simulink model "v3_sim_sf_sigma_r"  (R2023b)
settings: Solver=VariableStepAuto  StartTime=0.0  StopTime=100  RelTol=1e-10
libraries: simulink x2
settings Model: Creator=kiraa  LastModifiedBy=kiraa

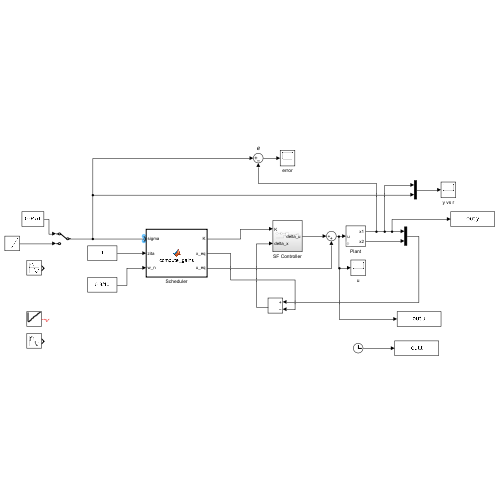
[thumbnail: Simulink's stored preview of the top-level diagram]
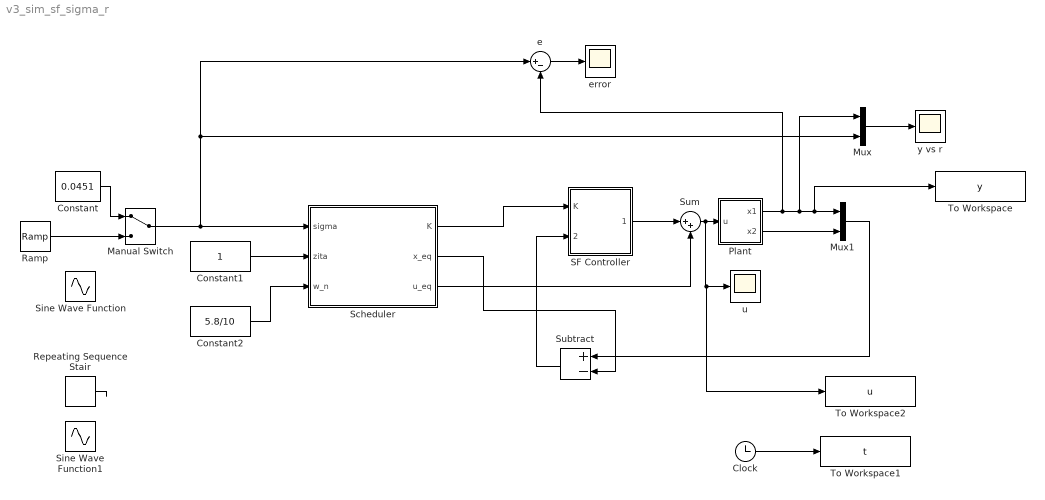
== system v3_sim_sf_sigma_r ==
  Clock : Clock
  Constant : Constant  Value=0.0451
  Constant1 : Constant
  Constant2 : Constant  Value=5.8/10
  Manual Switch : ManualSwitch
  Mux : Mux  Inputs=2
  Mux1 : Mux  Inputs=2
  Plant : Subsystem  mask{x1_0=0.1, x2_0=0}
      mask prompts: x1_0 "x1(0) [g/l]"; x2_0 "x2(0) [min^-1]"
  Ramp : simulink/Sources/Ramp  slope=-0.0005  start=0  InitialOutput=0.1
  Repeating Sequence Stair : simulink/Sources/Repeating Sequence Stair  OutValues=[0.1 0.2 0.3 0.4 0.5 0.6 0.7 0.8 0.9].'  tsamp=20  OutMin=[]  OutMax=[]  OutDataTypeStr=double  OutputDataTypeScalingMode=double  OutDataType=fixdt(0,8)  ConRadixGroup=Best Precision: Vector-wise  OutScaling=2^-12
  SF Controller : Subsystem
  Scheduler : MATLAB Function  TreatAsAtomicUnit=on
  Sine Wave Function : Sin  Amplitude=0.02  Bias=0.05  Frequency=0.1  SampleTime=0
  Sine Wave Function1 : Sin  Amplitude=0.001  Bias=0.0451  Frequency=0.1  Samples=1  SampleTime=2
  Subtract : Sum  Inputs=+-
  Sum : Sum  Inputs=|++
  To Workspace : ToWorkspace  VariableName=y  SampleTime=-1
  To Workspace1 : ToWorkspace  VariableName=t  SampleTime=-1
  To Workspace2 : ToWorkspace  VariableName=u  SampleTime=-1
  e : Sum  Inputs=|+-
  error : Scope
  u : Scope
  y vs r : Scope
  wires:
  Plant/1(x1) -> To Workspace/1, Mux1/1, Mux/1, e/2
  Mux/1 -> y vs r/1
  Constant/1 -> Manual Switch/1
  Manual Switch/1 -> Mux/2, e/1, Scheduler/1(sigma)
  SF Controller/1(delta_u) -> Sum/1
  e/1 -> error/1
  Sum/1 -> To Workspace2/1, u/1, Plant/1(u)
  Scheduler/3(u_eq) -> Sum/2
  Scheduler/1(K) -> SF Controller/1(K)
  Subtract/1 -> SF Controller/2(delta_x)
  Plant/2(x2) -> Mux1/2
  Mux1/1 -> Subtract/1
  Scheduler/2(x_eq) -> Subtract/2
  Constant2/1 -> Scheduler/3(w_n)
  Constant1/1 -> Scheduler/2(zita)
  Repeating Sequence Stair/1 -> ?
  Clock/1 -> To Workspace1/1
  Ramp/1 -> Manual Switch/2

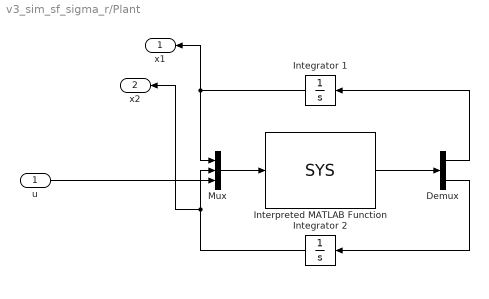
== system v3_sim_sf_sigma_r/Plant ==
  u : Inport
  Demux : Demux  Outputs=2
  Integrator 1 : Integrator  InitialCondition=x1_0
  Integrator 2 : Integrator  InitialCondition=x2_0
  Interpreted MATLAB Function : MATLABFcn  MATLABFcn=SYS  OutputDimensions=2
  Mux : Mux  Inputs=3
  x1 : Outport
  x2 : Outport  Port=2
  wires:
  Integrator 1/1 -> x1/1, Mux/1
  Demux/1 -> Integrator 1/1
  Mux/1 -> Interpreted MATLAB Function/1
  Integrator 2/1 -> x2/1, Mux/2
  Interpreted MATLAB Function/1 -> Demux/1
  Demux/2 -> Integrator 2/1
  u/1 -> Mux/3

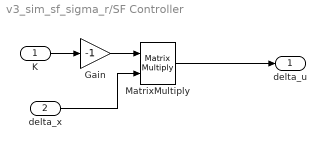
== system v3_sim_sf_sigma_r/SF Controller ==
  K : Inport
  delta_x : Inport  Port=2
  Gain : Gain  Gain=-1
  MatrixMultiply : Product  Multiplication=Matrix(*)
  delta_u : Outport
  wires:
  K/1 -> Gain/1
  Gain/1 -> MatrixMultiply/1
  delta_x/1 -> MatrixMultiply/2
  MatrixMultiply/1 -> delta_u/1

== matlab function v3_sim_sf_sigma_r/Scheduler ==
  data: sigma input; K output; x_eq output; u_eq output; zita input; w_n input
function [K,x_eq,u_eq] = compute_gains(sigma, zita, w_n)
    k1 = -(625*(20769187434139310514121985316880384*sigma^2*w_n^2 - 608412576695676974541561223184384*zita*sigma*w_n + 4455709505430790413433498137721))/(125913198819469569991864535983587328*sigma^3);
    k2 = -(2819253366733930496*sigma - 180143985094819840000*sigma*w_n*zita + 1319284474841913125)/(873698327709876224*sigma);
    K = [k1 k2];
    u_eq = -(399496308545527218176*sigma - 412936040625518808125)/(8736983277098762240000*sigma);
    x_eq = [sigma; -(1360087087465889792*sigma - 1319284474841913125)/(90071992547409920000*sigma)];
end
